simulink model "chap03_varsize_line_mdl"  (R2013b)
settings: Solver=ode4  StartTime=0.0  StopTime=10.0  FixedStep=0.01  RelTol=1e-3
settings Model: Creator=Administrator  LastModifiedBy=sunzx.fnst
settings DataIOCC: SaveFormat=Structure  SignalLogging=off
settings DebuggingCC: UnderspecifiedInitializationDetection=Simplified

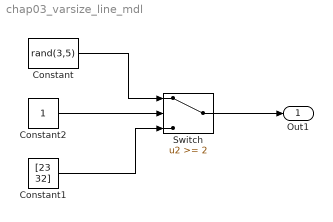
== system chap03_varsize_line_mdl ==
  Constant : Constant  Value=rand(3,5)
  Constant1 : Constant  Value=[23 32]
  Constant2 : Constant
  Switch : Switch  Threshold=2  AllowDiffInputSizes=on
  Out1 : Outport
  wires:
  Constant/1 -> Switch/1
  Constant1/1 -> Switch/3
  Switch/1 -> Out1/1
  Constant2/1 -> Switch/2
